simulink library "NullEventsBus"  (R2018b)
settings: Solver=VariableStepAuto  StartTime=0.0  StopTime=10.0  RelTol=1e-3
settings Model: Creator=RA24876  LastModifiedBy=RA24876
settings SFSimCC: SimUseLocalCustomCode=off
settings RTWCC: RTWUseLocalCustomCode=off
settings CodeAppCC: StateflowObjectComments=on

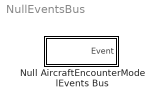
== system NullEventsBus ==
  Null AircraftEncounterModelEvents Bus : Subsystem  mask(Null AircraftEncounterModelEvents Bus){}
      mask help: Creates an AircraftEncounterModelEvents bus signal with all null values. Assign values to elements with a Bus Assignment block.

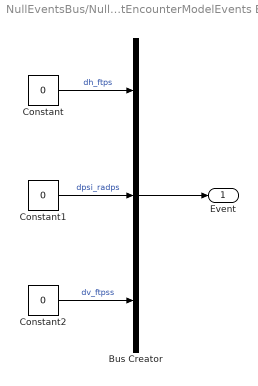
== system NullEventsBus/Null AircraftEncounterModelEvents Bus ==
  Bus Creator : BusCreator  Inputs=3  OutDataTypeStr=Bus: AircraftEncounterModelEvents
      settings: InheritFromInputs=off
  Constant : Constant  Value=0
  Constant1 : Constant  Value=0
  Constant2 : Constant  Value=0
  Event : Outport  OutDataTypeStr=Bus: AircraftEncounterModelEvents
  wires:
  Bus Creator/1 -> Event/1
  Constant2/1 -> Bus Creator/3  "dv_ftpss"
  Constant1/1 -> Bus Creator/2  "dpsi_radps"
  Constant/1 -> Bus Creator/1  "dh_ftps"
